simulink model "Image"  (R2016a)
settings: Solver=VariableStepAuto  StartTime=0.0  StopTime=10.0  RelTol=1e-3
libraries: visionsources x1, visionconversions x1, visionanalysis x1
settings Model: Creator=YLCB  LastModifiedBy=Ds

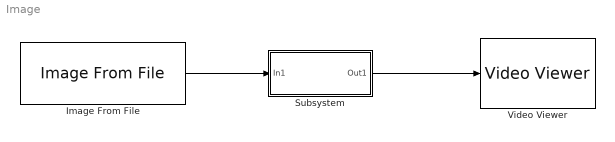
== system Image ==
  Image From File : visionsources/Image From File  Tag=vipblks_nd  FileName=E:\escritorio\Significados\ruidisimo.jpg  imagePorts=One multidimensional signal  Ts=inf  ImageDataType=Inherit from input image  Signed=on  WordLength=16  sdImageDataType=uint(8)  FractionLengthMode=User-defined  FractionLength=15  OutPortLabels=R|G|B
  Subsystem : Subsystem
  Video Viewer : VideoViewer  FigPos=[1 726 1366 626]
  wires:
  Image From File/1 -> Subsystem/1(In1)
  Subsystem/1(Out1) -> Video Viewer/1

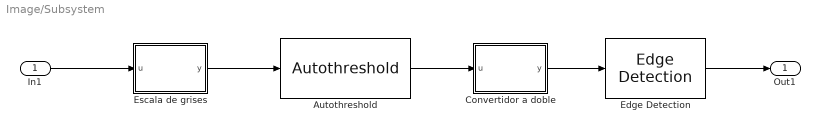
== system Image/Subsystem ==
  In1 : Inport
  Autothreshold : visionconversions/Autothreshold  operator=>  threshOut=off  effMetricOut=off  userDefinedRange=off  umin=0  umax=255  outOfRngOpt=Warn and saturate  scaleThreshold=off  scaleFactor=1  P1Mode=Specify word length  P1WordLength=32  P1FracLength=30  P2Mode=Specify word length  P2WordLength=32  P2FracLength=22  P3Mode=Specify word length  P3WordLength=32  P3FracLength=14  P4Mode=Binary point scaling  P4WordLength=32  P4FracLength=15  Q1Mode=Specify word length  Q1WordLength=32  Q1FracLength=16  EMMode=Specify word length  EMWordLength=16  EMFracLength=14  roundingMode=Floor  overflowMode=off
  "Convertidor a doble " : MATLAB Function  TreatAsAtomicUnit=on
  Edge Detection : visionanalysis/Edge Detection  method=Sobel  outputType=Binary image  userDefinedThreshold=off  thresholdSource=Input port  threshold=20  thresholdTuning=4  edgeThinning=off  threshold_canny=[0.25 0.60]  autoPercent=70  sigma=1  prodOutputMode=Binary point scaling  prodOutputWordLength=32  prodOutputFracLength=8  roundingMode=Floor  overflowMode=off
  "Escala de grises " : MATLAB Function  TreatAsAtomicUnit=on
  Out1 : Outport
  wires:
  In1/1 -> "Escala de grises "/1(u)
  Edge Detection/1 -> Out1/1
  "Escala de grises "/1(y) -> Autothreshold/1
  Autothreshold/1 -> "Convertidor a doble "/1(u)
  "Convertidor a doble "/1(y) -> Edge Detection/1

== matlab function Image/Subsystem/Convertidor a doble  ==
  data: u input; y output
function y = fcn(u)
%#codegen
y = double(u);

== matlab function Image/Subsystem/Escala de grises  ==
  data: u input; y output
function y = fcn(u)
%#codegen
Imggray=rgb2gray(u);
a=fspecial('gaussian');
gl1=imfilter(Imggray,a);
y = gl1;
